simulink model "Mdl_LPVOLtest"  (R2021b)
settings: Solver=FixedStepAuto  StartTime=0.0  StopTime=10.0  FixedStep=DT  RelTol=1e-3
values from neighbouring files (symbols this model uses):
  Drivetrain = 0.944    [DD_LPV.sldd]    (also in DD_Mdl.sldd)
  Ng = 97.0    [DD_LPV.sldd]    (also in DD_Mdl.sldd)
  OutList = <binary blob, 363 chars, not shown>    [DD_LPV.sldd]
undefined symbols (not defined in the file or in its folder): strmatch, sys12d_w
libraries: cstblocks x1
settings Model: DataDictionary=DD_LPV.sldd  Creator=ditt_aj  LastModifiedBy=ditt_aj
settings SolverCC: AlgebraicLoopSolver=TrustRegion
settings DebuggingCC: SFMachineParentedDataDiag=warning
settings SFSimCC: CustomCodeUndefinedFunction=UseInterfaceOnly

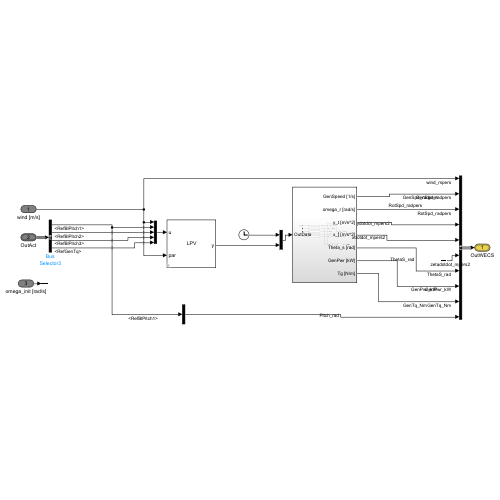
[thumbnail: Simulink's stored preview of the top-level diagram]
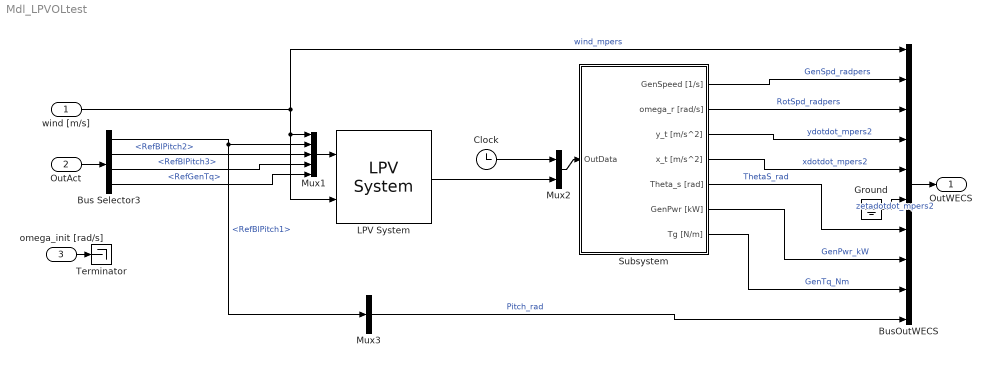
== system Mdl_LPVOLtest ==
  wind [m/s] : Inport
  OutAct : Inport  Port=2  OutDataTypeStr=Bus: slBus2
  omega_init [rad/s] : Inport  Port=3
  Bus Selector3 : BusSelector  OutputSignals=RefBlPitch1,RefBlPitch2,RefBlPitch3,RefGenTq
  BusOutWECS : BusCreator  Inputs=10  OutDataTypeStr=Bus: slBus1
  Clock : Clock
  Ground : Ground
  LPV System : cstblocks/Linear Parameter Varying/LPV System  sys=sysd  x0=x0  uOffset=uoff  yOffset=yoff  xOffset=xoff  opEquilOption=on  dxOffset=0  sysFixedOption=Use the first model in state-space array  sysFixed=sys12d_w(:,:,4)  AFixed=false  BFixed=false  CFixed=false  DFixed=false  uDelayFixed=false  yDelayFixed=false  iDelayFixed=false  IMethod=Nearest  EMethod=Clip  IndexSearch=Binary search  IndexBegin=on  OutputX=off  OutputXdot=off  OutputLTI=off  OutputOP=off  DataType=double  SimMode=Interpreted execution  InitBufferSize=1024  FixedBuffer=off
      settings: SourceProductBaseCode=CT
  Mux1 : Mux  Inputs=5
  Mux2 : Mux  Inputs=2
  Mux3 : Mux  Inputs=1
  Subsystem : Subsystem
  Terminator : Terminator
  OutWECS : Outport  OutDataTypeStr=Bus: slBus1
  wires:
  Mux1/1 -> LPV System/1
  Clock/1 -> Mux2/1
  LPV System/1 -> Mux2/2
  Mux2/1 -> Subsystem/1(OutData)
  OutAct/1 -> Bus Selector3/1
  Subsystem/3(y_t [m/s^2]) -> BusOutWECS/4  "ydotdot_mpers2"
  Subsystem/6(GenPwr [kW]) -> BusOutWECS/8  "GenPwr_kW"
  Subsystem/2(omega_r [rad/s]) -> BusOutWECS/3  "RotSpd_radpers"
  Bus Selector3/1 -> Mux3/1, Mux1/2  "<RefBlPitch1>"
  BusOutWECS/1 -> OutWECS/1
  Subsystem/5(Theta_s [rad]) -> BusOutWECS/7  "ThetaS_rad"
  wind [m/s]/1 -> BusOutWECS/1, LPV System/2, Mux1/1  "wind_mpers"
  Subsystem/1(GenSpeed [1/s]) -> BusOutWECS/2  "GenSpd_radpers"
  Subsystem/7(Tg [N/m]) -> BusOutWECS/9  "GenTq_Nm"
  Subsystem/4(x_t [m/s^2]) -> BusOutWECS/5  "xdotdot_mpers2"
  Ground/1 -> BusOutWECS/6  "zetadotdot_mpers2"
  Bus Selector3/4 -> Mux1/5  "<RefGenTq>"
  Bus Selector3/3 -> Mux1/4  "<RefBlPitch3>"
  Bus Selector3/2 -> Mux1/3  "<RefBlPitch2>"
  Mux3/1 -> BusOutWECS/10  "Pitch_rad"
  omega_init [rad/s]/1 -> Terminator/1

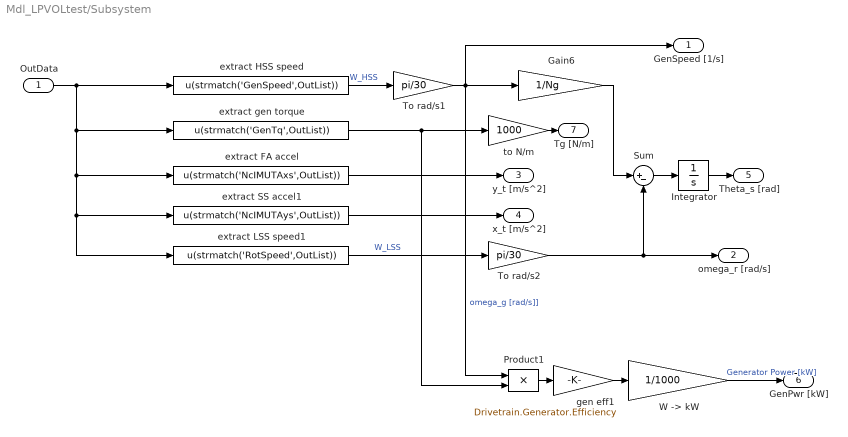
== system Mdl_LPVOLtest/Subsystem ==
  OutData : Inport
  Gain6 : Gain  Gain=1/Ng
  Integrator : Integrator
  Product1 : Product  RndMeth=Zero
  Sum : Sum  Inputs=|+-
  To rad/s1 : Gain  Gain=pi/30
  To rad/s2 : Gain  Gain=pi/30
  "W -> kW" : Gain  Gain=1/1000
  extract FA accel : Fcn  Expr=u(strmatch('NcIMUTAxs',OutList))
  extract HSS speed : Fcn  Expr=u(strmatch('GenSpeed',OutList))
  extract LSS speed1 : Fcn  Expr=u(strmatch('RotSpeed',OutList))
  extract SS accel1 : Fcn  Expr=u(strmatch('NcIMUTAys',OutList))
  extract gen torque : Fcn  Expr=u(strmatch('GenTq',OutList))
  gen eff1 : Gain  Gain=Drivetrain.Generator.Efficiency
  to N/m : Gain  Gain=1000
  GenSpeed [1/s] : Outport  VectorParamsAs1DForOutWhenUnconnected=off
  omega_r [rad/s] : Outport  Port=2  VectorParamsAs1DForOutWhenUnconnected=off
  y_t [m/s^2] : Outport  Port=3  VectorParamsAs1DForOutWhenUnconnected=off
  x_t [m/s^2] : Outport  Port=4  VectorParamsAs1DForOutWhenUnconnected=off
  Theta_s [rad] : Outport  Port=5  VectorParamsAs1DForOutWhenUnconnected=off
  GenPwr [kW] : Outport  Port=6  VectorParamsAs1DForOutWhenUnconnected=off
  Tg [N/m] : Outport  Port=7  VectorParamsAs1DForOutWhenUnconnected=off
  wires:
  to N/m/1 -> Tg [N/m]/1
  OutData/1 -> extract HSS speed/1, extract gen torque/1, extract LSS speed1/1, extract SS accel1/1, extract FA accel/1
  extract FA accel/1 -> y_t [m/s^2]/1
  extract HSS speed/1 -> To rad/s1/1  "W_HSS"
  extract SS accel1/1 -> x_t [m/s^2]/1
  extract LSS speed1/1 -> To rad/s2/1  "W_LSS"
  Gain6/1 -> Sum/1
  To rad/s2/1 -> Sum/2, omega_r [rad/s]/1
  Sum/1 -> Integrator/1
  Integrator/1 -> Theta_s [rad]/1
  "W -> kW"/1 -> GenPwr [kW]/1  "Generator Power [kW]"
  gen eff1/1 -> "W -> kW"/1
  Product1/1 -> gen eff1/1
  To rad/s1/1 -> Product1/1, Gain6/1, GenSpeed [1/s]/1  "omega_g [rad/s]]"
  extract gen torque/1 -> Product1/2, to N/m/1
